simulink model "Task1"  (R2019b)
settings: Solver=VariableStepAuto  StartTime=0.0  StopTime=10.0  RelTol=1e-3
settings Model: Creator=12393  LastModifiedBy=12393

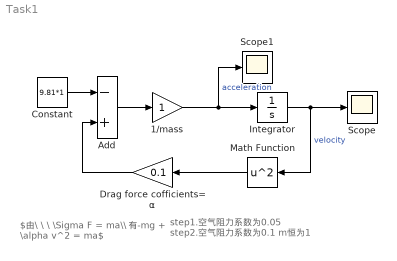
== system Task1 ==
  note: step1.空气阻力系数为0.05
      | step2.空气阻力系数为0.1
      | m恒为1
  note: $由\ \ \ \Sigma F = ma\\ 有-mg + \alpha v^2 = ma$
  "1/mass " : Gain
  Add : Sum  Inputs=-+
  Constant : Constant  Value=9.81*1
  Drag force cofficients=α : Gain  Gain=0.1
  Integrator : Integrator
  Math Function : Math  Operator=square  SignedPower=off  SaturateOnIntegerOverflow=on
  Scope : Scope
  Scope1 : Scope
  wires:
  Constant/1 -> Add/1
  Add/1 -> "1/mass "/1
  "1/mass "/1 -> Scope1/1, Integrator/1  "acceleration"
  Integrator/1 -> Math Function/1, Scope/1  "velocity"
  Math Function/1 -> Drag force cofficients=α/1
  Drag force cofficients=α/1 -> Add/2
